simulink model "Sim_Multi"  (R2023a)
settings: Solver=FixedStepAuto  StartTime=0.0  StopTime=20  FixedStep=t_sim  MaxStep=t_control  RelTol=1e-5  EnableMultiTasking=on
InitFcn:
  | %--------------------------------------------------------------------------
  | %% Multirotor Dynamic Simulation Environment for the Testing of GNC Algorithms
  | % This simulation is part of the Master's thesis titled
  | % "A Modular Simulation Environment for the Improved Dynamic Simulation of
  | % Multirotor Unmanned Aerial Vehicles",
  | % submitted to the University of Illinois at Urbana-Champaign in May 2016.
  | % The thesis itself can be found here: http://hdl.handle.net/2142/90660
  | % Jan Vervoorst, vervoors@illinois.edu
  | % University of Illinois 2015/16
  | %--------------------------------------------------------------------------
  | %% Initialization routine for the Simulink simulation file Sim_Multi.slx
  | %--------------------------------------------------------------------------
  | clear all;close all;clc
  | %--------------------------------------------------------------------------
  | t_control = 1/500;          % Controller/state estimation frequency 500Hz [s]
  | t_sim = t_control/2;        % Simulation frequency 1000Hz [s]
  | sim_time = 10.0;            % Duration of simulation [sec]
  | r2d = 180/pi;               % Conversion factor radians to degrees [deg/rad]
  | d2r = pi/180;               % Conversion factor degrees to radians [rad/deg]
  | g = 9.80665;                % Acceleration of gravity [m/s^2]
  | rpm2radpersec = 2*pi/60;    % Conversion factor RPM to rad/sec [rad/(s*rpm)]
  | rho = 1.225;                % Density of air [kg/m^3]
  | %--------------------------------------------------------------------------
  | %%%%%%%%%%%%%%%%%%%%%%%%%%%%%%%%%%%%%%%%%%%%%%%%%%%%%%%%%%%%%%%%%%%%%%%%%%%
  | %               Quad specific configuration parameters                    %
  | %%%%%%%%%%%%%%%%%%%%%%%%%%%%%%%%%%%%%%%%%%%%%%%%%%%%%%%%%%%%%%%%%%%%%%%%%%%
  | % The coordinate system used in this model is defined as follows:
  | % X: pointing forward, Roll axis
  | % Y: pointing to the right, Pitch axis
  | % Z: pointing down, Yaw axis
  | % To define the geometry of the airframe, the following convention is used:
  | % - the base airframe is assumed to be somewhat symmetric
  | % - the CoG for the base airframe coincides with the geometric center in X/Y plane (but is shifted along Z axis)
  | % - the motor arm length in X/Y plane is defined as the distance to the geometric center of the base airframe
  | % - motor thrust is generated at the prop, which is offset a distance (along Z) from the geometric center
  | % - motor thrust vector may be misaligned from purely Z direction, so a set of rotation angles is given for each motor
  | % - real position of CoG is given as a position vector from geometric center
  | % - everything is expressed in body coordinate system described above
  | %%%%%%%%%%%%%%%%%%%%%%%%%%%%%%%%%%%%%%%%%%%%%%%%%%%%%%%%%%%%%%%%%%%%%%%%%%%
  | Noise_flag = 0;                 % Set to 1 for sensor/estimation noise, to 0 for no noise
  | Coriolis_correction = 1;        % Set to 1 to cancel omega x (J*omega) term in control law, 0 if not
  | Dyn_thrust = 1;                 % Set to 1 to engage dynamic thrust effects, to 0 to disengage
  | Blade_flapping = 1;             % Set to 1 to engage blade flapping effects, to 0 to disengage
  | %%%%%%%%%%%%%%%%%%%%%%%%%%%%%%%%
  | % Initial conditions
  | Att_init = [0;0;0] * d2r;       % Initial airframe attitude in Euler angles Roll/Pitch/Yaw for 6DOF block [deg]
  | omega_init = [0;0;0];           % Initial angular rates in Body frame for 6DOF block [rad/s]
  | Vb_init = [0;0;0];              % Initial velocity in Body frame for 6DOF block [m/s]
  | Xi_init = [0;0;0];              % Initial position in Inertial frame for 6DOF block [m]
  | rpm_init = 3104.5025852;        % Initial motor speed [rpm]
  | q_init = rpy2quat(Att_init);    % Compute the initial attitude quaternion
  | R_IB_init = rpy2rot(Att_init);  % Compute the initial rotation matrix R_IB
  | Vi_init = R_IB_init' * Vb_init; % Compute the initial velocity in Inertial axes
  | %%%%%%%%%%%%%%%%%%%%%%%%%%%%%%%%
  | % Parameters for aerodynamic drag computation
  | a = 0.060;                      % Surface area of airframe visible along the Body x axis [m^2]
  | b = 0.060;                      % Surface area of airframe visible along the Body y axis [m^2]
  | c = 0.060;                      % Surface area of airframe visible along the Body z axis [m^2]
  | C_D = 0.40;                     % Drag coefficient [dimensionless]
  | Surface_params = [a;b;c];       % Combine the surface area parameters
  | %%%%%%%%%%%%%%%%%%%%%%%%%%%%%%%%
  | % Parameters for dynamic thrust computation
  | v_h = 4.0;                      % Induced aerodynamic velocity at hover [m/s]
  | kappa = 1.00;                   % Value for induced power factor in hover (chosen to make transition from different states continuous)
  | k1 = -1.125;                    % Empirical values taken from Hoffmann_2011
  | k2 = -1.372;                    % Empirical values taken from Hoffmann_2011
  | k3 = -1.718;                    % Empirical values taken from Hoffmann_2011
  | k4 = -0.655;                    % Empirical values taken from Hoffmann_2011
  | %%%%%%%%%%%%%%%%%%%%%%%%%%%%%%%%
  | % Parameters for blade flapping computation
  | k_a1s = 1.5 / 4.0;              % Gain in linear relationship between wind velocity and flapping angle [deg/(m/s)]
  | k_beta = 0.23;                  % Stiffness of the propeller blades [Nm/rad]
  | %%%%%%%%%%%%%%%%%%%%%%%%%%%%%%%%
  | % Real airframe data
  | CoG_real = [0;0;0.001];         % Location of center of gravity w.r.t. geometric center (in Body axes) [m]
  | mass_real = 0.550;              % Complete airframe mass [kg]
  | Jxx = 0.003960;                 %
  | Jxy = 0;                        %
  | Jxz = 0;                        %
  | Jyx = 0;                        %
  | Jyy = 0.003845;                 % Moment of inertia for multirotor w.r.t center of gravity [kg*m^2]
  | Jyz = 0;                        %
  | Jzx = 0;                        %
  | Jzy = 0;                        %
  | Jzz = 0.007350;                 %
  | J_real = [Jxx Jxy Jxz;Jyx Jyy Jyz;Jzx Jzy Jzz]; % Moment of inertia matrix
  | %%%%%%%%%%%%%%%%%%%%%%%%%%%%%%%%
  | % MotorMatrix_real holds all the information about the actual performance
  | % of each actuator. The data is arranged as one row per motor/prop combo:
  | % 1      : Motor arm angle measured clockwise (looking from above) from the positive X axis (forward direction) [deg]
  | % 2      : Distance of prop/motor in X/Y plane from the geometric center of the airframe [m]
  | % 3      : Distance of prop/motor in Z direction from the geometric center of the airframe [m]
  | % 4      : Direction of prop rotation: -1 for CW, +1 for CCW [unitless]
  | % 5      : Control effectiveness of the actuator (nominally 1.0)
  | % 6      : First-order motor transfer function time constant [sec]
  | % 7..8   : Two coefficients that describe the RPM to thrust [N] transfer function for static conditions [a1 a2]
  | %          Thrust = a1 * RPM + a2 * RPM^2
  | % 9..10  : Two coefficients that describe the RPM to torque [Nm] transfer function for static conditions [b1 b2]
  | %          Torque = b1 * RPM + b2 * RPM^2
  | % 11     : Minimum RPM value of the actuator
  | % 12     : Maximum RPM value of the actuator
  | % 13..15 : Rotations of thrust vector around Body-fixed axes away from nominal direction [deg]
  | %          Nominal direction of thrust vector is [0;0;-1]
  | %          Rotation order from body to motor axes is Yaw/Pitch/Roll (Euler angle sequence (1,2,3))
  | % 16     : Propeller diameter [m]
  | % 17     : Propeller mass [kg]
  | 
  | length1 = 0.170;
  | length2 = 0.170;
  | length3 = 0.170;
  | length4 = 0.170;
  | 
  | MotorMatrix_real = [045 , length1 , -0.028 , -1 , 1.0 , 0.010 , [9.6820 , 0.010872]*1e-5 , [1.4504 , 0.0016312]*1e-6 , 0000 , 6000 , [0.0 , 0.0 , 0.0] , 8*2.54/100 , 11/1000; ...
  |                     135 , length2 , -0.028 , +1 , 1.0 , 0.010 , [9.6820 , 0.010872]*1e-5 , [1.4504 , 0.0016312]*1e-6 , 0000 , 6000 , [0.0 , 0.0 , 0.0] , 8*2.54/100 , 11/1000; ...
  |                     225 , length3 , -0.028 , -1 , 1.0 , 0.010 , [9.6820 , 0.010872]*1e-5 , [1.4504 , 0.0016312]*1e-6 , 0000 , 6000 , [0.0 , 0.0 , 0.0] , 8*2.54/100 , 11/1000; ...
  |                     315 , length4 , -0.028 , +1 , 1.0 , 0.010 , [9.6820 , 0.010872]*1e-5 , [1.4504 , 0.0016312]*1e-6 , 0000 , 6000 , [0.0 , 0.0 , 0.0] , 8*2.54/100 , 11/1000];
  | %%%%%%%%%%%%%%%%%%%%%%%%%%%%%%%%
  | % Nominal airframe data (without disturbance/uncertainties)
  | CoG_nominal = [0;0;0.001];      % Location of center of gravity w.r.t. geometric center (in Body axes) [m]
  | mass_nominal = 0.550;           % Complete airframe mass [kg]
  | Jxx = 0.003960;                 %
  | Jxy = 0;                        %
  | Jxz = 0;                        %
  | Jyx = 0;                        %
  | Jyy = 0.003845;                 % Moment of inertia for multirotor w.r.t center of gravity [kg*m^2]
  | Jyz = 0;                        %
  | Jzx = 0;                        %
  | Jzy = 0;                        %
  | Jzz = 0.007350;                 %
  | J_nominal = [Jxx Jxy Jxz;Jyx Jyy Jyz;Jzx Jzy Jzz]; % Moment of inertia matrix
  | k_torque = 3/200;               % Factor how thrust and induced moment are related (from motor test data)
  | thrust_reserve = 0.10;          % Limit total commanded thrust to 10...90% of max thrust to still allow maneuverability
  | %%%%%%%%%%%%%%%%%%%%%%%%%%%%%%%%
  | % MotorMatrix_nominal holds the nominal information that the controller
  | % assumes about each actuator. Again, the data is arranged as one row per
  | % motor/prop combo:
  | % 1      : Motor arm angle measured clockwise (looking from above) from the positive X axis (forward direction) [deg]
  | % 2      : Distance of prop/motor in X/Y plane from the geometric center of the airframe [m]
  | % 3      : Distance of prop/motor in Z direction from the geometric center of the airframe [m]
  | % 4      : Direction of prop rotation: -1 for CW, +1 for CCW [unitless]
  | % 5      : Control effectiveness of the actuator (nominally 1.0)
  | % 6      : First-order motor transfer function time constant [sec]
  | % 7..8   : Two coefficients that describe the RPM to thrust [N] transfer function for static conditions [a1 a2]
  | %          Thrust = a1 * RPM + a2 * RPM^2
  | % 9..10  : Two coefficients that describe the RPM to torque [Nm] transfer function for static conditions [b1 b2]
  | %          Torque = b1 * RPM + b2 * RPM^2
  | % 11     : Minimum RPM value of the actuator
  | % 12     : Maximum RPM value of the actuator
  | % 13..15 : Rotations of thrust vector around Body-fixed axes away from nominal direction [deg]
  | %          Nominal direction of thrust vector is [0;0;-1]
  | %          Rotation order from body to motor axes is Yaw/Pitch/Roll (Euler angle sequence (1,2,3))
  | % 16     : Propeller diameter [m]
  | % 17     : Propeller mass [kg]
  | MotorMatrix_nominal = [045 , length1 , -0.028 , -1 , 1.0 , 0.010 , [9.6820 , 0.010872]*1e-5 , [1.4504 , 0.0016312]*1e-6 , 0000 , 6000 , [0.0 , 0.0 , 0.0] , 8*2.54/100 , 11/1000; ...
  |                        135 , length2 , -0.028 , +1 , 1.0 , 0.010 , [9.6820 , 0.010872]*1e-5 , [1.4504 , 0.0016312]*1e-6 , 0000 , 6000 , [0.0 , 0.0 , 0.0] , 8*2.54/100 , 11/1000; ...
  |                        225 , length3 , -0.028 , -1 , 1.0 , 0.010 , [9.6820 , 0.010872]*1e-5 , [1.4504 , 0.0016312]*1e-6 , 0000 , 6000 , [0.0 , 0.0 , 0.0] , 8*2.54/100 , 11/1000; ...
  |                        315 , length4 , -0.028 , +1 , 1.0 , 0.010 , [9.6820 , 0.010872]*1e-5 , [1.4504 , 0.0016312]*1e-6 , 0000 , 6000 , [0.0 , 0.0 , 0.0] , 8*2.54/100 , 11/1000];
  | %%%%%%%%%%%%%%%%%%%%%%%%%%%%%%%%%%%%%%%%%%%%%%%%%%%%%%%%%%%%%%%%%%%%%%%%%%%
  | %                          Radio scaling factor                           %
  | %%%%%%%%%%%%%%%%%%%%%%%%%%%%%%%%%%%%%%%%%%%%%%%%%%%%%%%%%%%%%%%%%%%%%%%%%%%
  | % Compute the scaling factor to turn radio throttle command into a thrust value
  | max_thrust = 0;
  | min_thrust = 0;
  | for i = 1:size(MotorMatrix_nominal,1)
  |     max_thrust = max_thrust + (MotorMatrix_nominal(i,7)*MotorMatrix_nominal(i,12)+MotorMatrix_nominal(i,8)*MotorMatrix_nominal(i,12)^2);
  |     min_thrust = min_thrust + (MotorMatrix_nominal(i,7)*MotorMatrix_nominal(i,11)+MotorMatrix_nominal(i,8)*MotorMatrix_nominal(i,11)^2);
  | end
  | thrust_gain = (max_thrust - min_thrust) / 1000;
  | thrust_offset = min_thrust;
  | % %%%%%%%%%%%%%%%%%%%%%%%%%%%%%%%%%%%%%%%%%%%%%%%%%%%%%%%%%%%%%%%%%%%%%%%%%%%
  | % %                   Compute the motor mapping matrix                      %
  | % %%%%%%%%%%%%%%%%%%%%%%%%%%%%%%%%%%%%%%%%%%%%%%%%%%%%%%%%%%%%%%%%%%%%%%%%%%%
  | % % This matrix describes the mapping from body torques to motor thrusts.
  | for i = 1:size(MotorMatrix_nominal,1)
  |     % The vector from nominal center of gravity to nominal location of each propeller
  |     prop_vector(i,1:3) = [abs(MotorMatrix_nominal(i,2)) * [cos(MotorMatrix_nominal(i,1)*d2r);sin(MotorMatrix_nominal(i,1)*d2r)];MotorMatrix_nominal(i,3)] - CoG_nominal;
  |     % The nominal direction in which each motor generates thrust force
  |     thrust_direction(i,1:3) = -[cos(MotorMatrix_nominal(i,13)*d2r)*sin(MotorMatrix_nominal(i,14)*d2r)*cos(MotorMatrix_nominal(i,15)*d2r)+sin(MotorMatrix_nominal(i,13)*d2r)*sin(MotorMatrix_nominal(i,15)*d2r); ...
  |                               cos(MotorMatrix_nominal(i,13)*d2r)*sin(MotorMatrix_nominal(i,14)*d2r)*sin(MotorMatrix_nominal(i,15)*d2r)-sin(MotorMatrix_nominal(i,13)*d2r)*cos(MotorMatrix_nominal(i,15)*d2r); ...
  |                               cos(MotorMatrix_nominal(i,13)*d2r)*cos(MotorMatrix_nominal(i,14)*d2r)];
  |     % The B matrix relates motor thrust to body torques and thrust
  |     % Each column describes one motor/prop. Entries by row 1-4:
  |     % contributions to roll/pitch/yaw torques and thrust, respectively
  | 	B(1:3,i) = cross(prop_vector(i,:)',thrust_direction(i,:)') + k_torque*thrust_direction(i,:)'*MotorMatrix_nominal(i,4);
  |     B(4,i) = 1.0;
  | end
  | % For any airframe with a number of actuators other than four, the B matrix
  | % is nonsquare and therefore taking the regular inverse will not work.
  | % Instead we use the Moore-Penrose pseudoinverse for matrices with linearly
  | % independent rows:
  | MotorMap = B' * inv(B * B');
  | 
  | %%%%%%%%%%%%%%%%%%%%%%%%%%%%%%%%%%%%%%%%%%%%%%%%%%%%%%%%%%%%%%%%%%%%%%%%%%%
  | %              Tuning parameters for the controllers                      %
  | %%%%%%%%%%%%%%%%%%%%%%%%%%%%%%%%%%%%%%%%%%%%%%%%%%%%%%%%%%%%%%%%%%%%%%%%%%%
  | % Controller settings
  | Att_cmd_init = [0;0;0] * d2r;           % Initial attitude command for quaternion strapdown equation initialization in control law
  | MaxRate_cmd = [360;360;120] * d2r;      % Maximum rate command at full stick deflection [rad/s]
  | MaxAtt_cmd = 50 * d2r;                  % Max angle command at full stick deflection [rad]
  | Ref_bw = 10.0;                          % Reference system bandwidth for rate command generation in attitude control
  | %%%%%%%%%%%%%%%%%%%%%%%%%%%%%%%%
  | % Gains for simple PI controller on rates
  | Kp_1  = 15*[1;1;1.5];
  | Ki_1  = 10*[1;1;1.5];
  | Kff_1 = 0.7*[1;1;0.95];
undefined symbols (not defined in the file or in its folder): DiscIntNeverNeededParam, rpy2quat, thrust2rpm
libraries: simulink x20
(part 1 of 4)
settings Model: Creator=JV  LastModifiedBy=divij
settings SolverCC: AlgebraicLoopSolver=TrustRegion
settings DataIOCC: LimitDataPoints=on  SaveFormat=Structure  SignalLoggingSaveFormat=ModelDataLogs  ReturnWorkspaceOutputs=off
settings OptimizationCC: DefaultParameterBehavior=Inlined  UseDivisionForNetSlopeComputation=on  GainParamInheritBuiltInType=on  UseFloatMulNetSlope=on  InlineInvariantSignals=on  ExpressionDepthLimit=2147483647  ZeroExternalMemoryAtStartup=off  ZeroInternalMemoryAtStartup=off  EfficientFloat2IntCast=on  LifeSpan=1  OptimizeDataStoreBuffers=off  BusAssignmentInplaceUpdate=off
settings DebuggingCC: UnderspecifiedInitializationDetection=Classic  SolverPrmCheckMsg=warning  FcnCallInpInsideContextMsg=warning  UnconnectedInputMsg=warning  UnconnectedOutputMsg=warning  UnconnectedLineMsg=warning  StateNameClashWarn=warning  SFUnexpectedBacktrackingDiag=warning  SFNoUnconditionalDefaultTransitionDiag=warning  SFExecutionAtInitializationDiag=none  ArithmeticOperatorsInVariantConditions=warning
settings HardwareCC: ProdBitPerPointer=32  ProdBitPerSizeT=32  ProdBitPerPtrDiffT=32  ProdLargestAtomicFloat=None  ProdIntDivRoundTo=Undefined  ProdEndianess=Unspecified  ProdWordSize=32  ProdHWDeviceType=32-bit Generic
settings ModelReferenceCC: EnableRefExpFcnMdlSchedulingChecks=on  PropagateSignalLabelsOutOfModel=off
settings SFSimCC: SimUseLocalCustomCode=off  MATLABDynamicMemAlloc=off  CustomCodeUndefinedFunction=UseInterfaceOnly
settings RTWCC: PackageGeneratedCodeAndArtifacts=on  GenerateReport=on  RTWUseLocalCustomCode=off  Toolchain=Catkin  BuildConfiguration=Debug  LaunchReport=on  TargetLang=C++
settings CodeAppCC: ForceParamTrailComments=on  EnableCustomComments=on
settings GRTTargetCC: TargetLangStandard=C++11 (ISO)  CombineSignalStateStructs=on  MatFileLogging=off  CodeInterfacePackaging=C++ class  SupportVariableSizeSignals=on  MultiInstanceErrorCode=Warning
settings ConfigComp: CovMetricSettings=dw  CovSaveCumulativeToWorkspaceVar=on  CovSaveSingleToWorkspaceVar=on  CovExternalEMLEnable=off  CovSFcnEnable=off

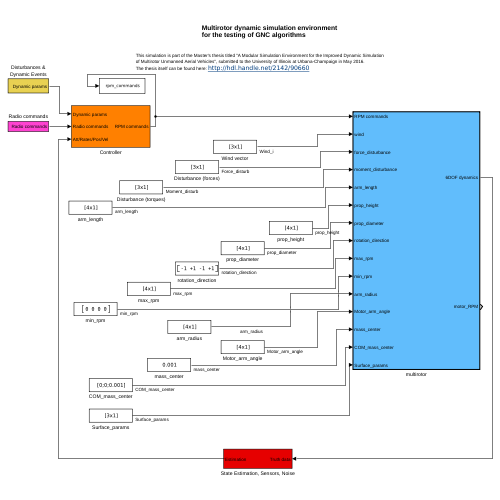
[thumbnail: Simulink's stored preview of the top-level diagram]
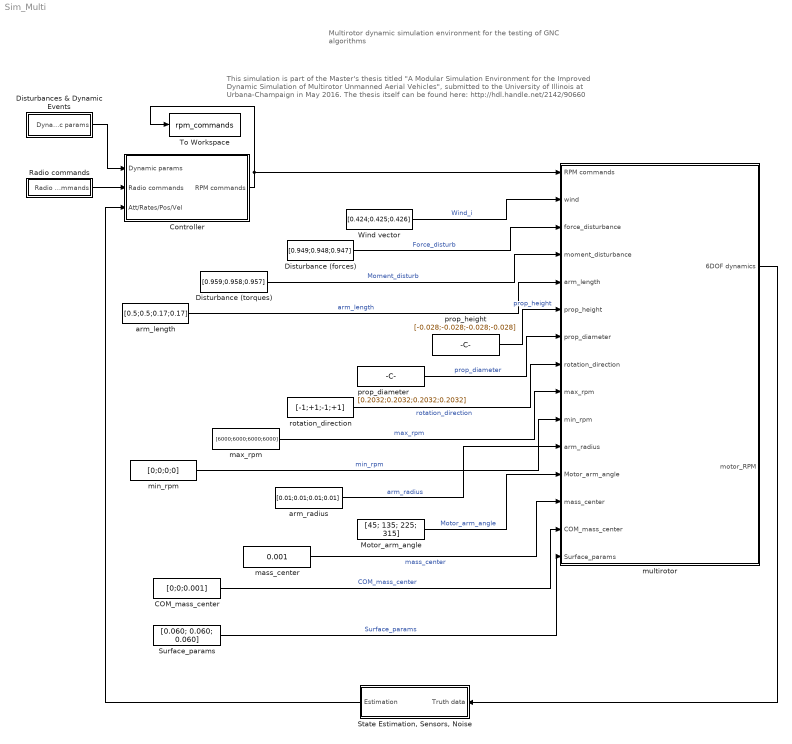
== system Sim_Multi ==
  note: This simulation is part of the Master's thesis titled "A Modular Simulation Environment for the Improved Dynamic Simulation
      | of Multirotor Unmanned Aerial Vehicles", submitted to the University of Illinois at Urbana-Champaign in May 2016.
      | The thesis itself can be found here: http://hdl.handle.net/2142/90660
  note: Multirotor dynamic simulation environment
      | for the testing of GNC algorithms
  COM_mass_center : Constant  Value=[0;0;0.001]
  Controller : Subsystem
  Disturbance (forces) : Constant  Value=[0.949;0.948;0.947]
  Disturbance (torques) : Constant  Value=[0.959;0.958;0.957]
  Disturbances & Dynamic Events : Subsystem
  Motor_arm_angle : Constant  Value=[45; 135; 225; 315]
  Radio commands : Subsystem
  "State Estimation, Sensors, Noise" : Subsystem
  Surface_params : Constant  Value=[0.060; 0.060; 0.060]
  To Workspace : ToWorkspace  VariableName=rpm_commands  SaveFormat=Structure  SampleTime=-1
      settings: Save2DSignal=2-D array (concatenate along first dimension)
  Wind vector : Constant  Value=[0.424;0.425;0.426]
  arm_length : Constant  Value=[0.5;0.5;0.17;0.17]
  arm_radius : Constant  Value=[0.01;0.01;0.01;0.01]
  mass_center : Constant  Value=0.001
  max_rpm : Constant  Value=[6000;6000;6000;6000]
  min_rpm : Constant  Value=[0;0;0;0]
  multirotor : Subsystem  TreatAsAtomicUnit=on
  prop_diameter : Constant  Value=[0.2032;0.2032;0.2032;0.2032]
  prop_height : Constant  Value=[-0.028;-0.028;-0.028;-0.028]
  rotation_direction : Constant  Value=[-1;+1;-1;+1]
  wires:
  multirotor/1(6DOF dynamics) -> "State Estimation, Sensors, Noise"/1(Truth data)
  Radio commands/1(Radio commands) -> Controller/2(Radio commands)
  "State Estimation, Sensors, Noise"/1(Estimation) -> Controller/3(Att/Rates/Pos/Vel)
  Disturbances & Dynamic Events/1(Dynamic params) -> Controller/1(Dynamic params)
  Controller/1(RPM commands) -> To Workspace/1, multirotor/1(RPM commands)
  Wind vector/1 -> multirotor/2(wind)  "Wind_i"
  Disturbance (forces)/1 -> multirotor/3(force_disturbance)  "Force_disturb"
  Disturbance (torques)/1 -> multirotor/4(moment_disturbance)  "Moment_disturb"
  arm_length/1 -> multirotor/5(arm_length)  "arm_length"
  prop_height/1 -> multirotor/6(prop_height)  "prop_height"
  prop_diameter/1 -> multirotor/7(prop_diameter)  "prop_diameter"
  rotation_direction/1 -> multirotor/8(rotation_direction)  "rotation_direction"
  max_rpm/1 -> multirotor/9(max_rpm)  "max_rpm"
  min_rpm/1 -> multirotor/10(min_rpm)  "min_rpm"
  arm_radius/1 -> multirotor/11(arm_radius)  "arm_radius"
  Motor_arm_angle/1 -> multirotor/12(Motor_arm_angle)  "Motor_arm_angle"
  mass_center/1 -> multirotor/13(mass_center)  "mass_center"
  COM_mass_center/1 -> multirotor/14(COM_mass_center)  "COM_mass_center"
  Surface_params/1 -> multirotor/15(Surface_params)  "Surface_params"

== system Sim_Multi/Controller ==
  note: All system parameters used in this block are the nominal parameters
      | that the controller is given about the system.
      | The true parameters of the dynamic system such as mass, inertia,
      | motor mapping matrix, ... may differ from these values.
  Dynamic params : Inport
  Radio commands : Inport  Port=2
  Att/Rates/Pos/Vel : Inport  Port=3
  Controller Structure : Subsystem
  Mapping thrust to rpm and saturation : Subsystem
  Motor mapping : Subsystem
  Reshape : Reshape  OutputDimensionality=Column vector (2-D)
  RPM commands : Outport
  tag scope: RPM_commands=global
  wires:
  Att/Rates/Pos/Vel/1 -> Controller Structure/2(Att/Rates/Pos/Vel)
  Controller Structure/1(Torques/thrust cmd) -> Motor mapping/1(Torques/thrust cmd)
  Radio commands/1 -> Controller Structure/1(Radio commands)
  Reshape/1 -> RPM commands/1
  Dynamic params/1 -> Controller Structure/3(Dynamic params), Mapping thrust to rpm and saturation/2(Dynamic parameters)
  Mapping thrust to rpm and saturation/1(RPM_cmd) -> [RPM_commands], Reshape/1
  Motor mapping/1(Thrust cmds) -> Mapping thrust to rpm and saturation/1(Thrust_cmds)

== system Sim_Multi/Disturbances & Dynamic Events ==
  Bus Creator : BusCreator  Inputs=12
  Constant : Constant  Value=MotorMatrix_real
  Constant1 : Constant  Value=CoG_real
  Constant2 : Constant  Value=mass_real
  Constant3 : Constant  Value=J_real
  Constant4 : Constant  Value=MotorMatrix_nominal
  Constant5 : Constant  Value=CoG_nominal
  Constant6 : Constant  Value=mass_nominal
  Constant7 : Constant  Value=J_nominal
  Disturbance (forces) : Constant  Value=0*[1;1;1]
  Disturbance (torques) : Constant  Value=0*[1;1;1]
  Surface area params : Constant  Value=Surface_params
  Wind vector : Constant  Value=[0;0;0]
  Dynamic params : Outport
  wires:
  Bus Creator/1 -> Dynamic params/1
  Constant/1 -> Bus Creator/1  "MotorMatrix_real"
  Constant1/1 -> Bus Creator/2  "CoG_real"
  Constant2/1 -> Bus Creator/3  "mass_real"
  Constant3/1 -> Bus Creator/4  "J_real"
  Surface area params/1 -> Bus Creator/12  "Surface_params"
  Disturbance (torques)/1 -> Bus Creator/11  "Moment_disturb"
  Disturbance (forces)/1 -> Bus Creator/10  "Force_disturb"
  Wind vector/1 -> Bus Creator/9  "Wind_i"
  Constant4/1 -> Bus Creator/5  "MotorMatrix_nominal"
  Constant5/1 -> Bus Creator/6  "CoG_nominal"
  Constant6/1 -> Bus Creator/7  "mass_nominal"
  Constant7/1 -> Bus Creator/8  "J_nominal"

== system Sim_Multi/Radio commands ==
  Rate Transition : RateTransition  OutPortSampleTime=t_control
  Rate commands : Subsystem
  Radio commands : Outport
  wires:
  Rate commands/1(Rate commands) -> Rate Transition/1
  Rate Transition/1 -> Radio commands/1

== system Sim_Multi/State Estimation, Sensors, Noise ==
  Truth data : Inport
  Rate Transition : RateTransition  OutPortSampleTime=t_control
  Sensor models : Subsystem
  State estimation : Subsystem
  Estimation : Outport
  wires:
  State estimation/1(Att/Pos/Vel/Accel) -> Rate Transition/1
  Sensor models/1(Corrupted) -> State estimation/1(Sensors)
  Truth data/1 -> Sensor models/1(Truth)
  Rate Transition/1 -> Estimation/1

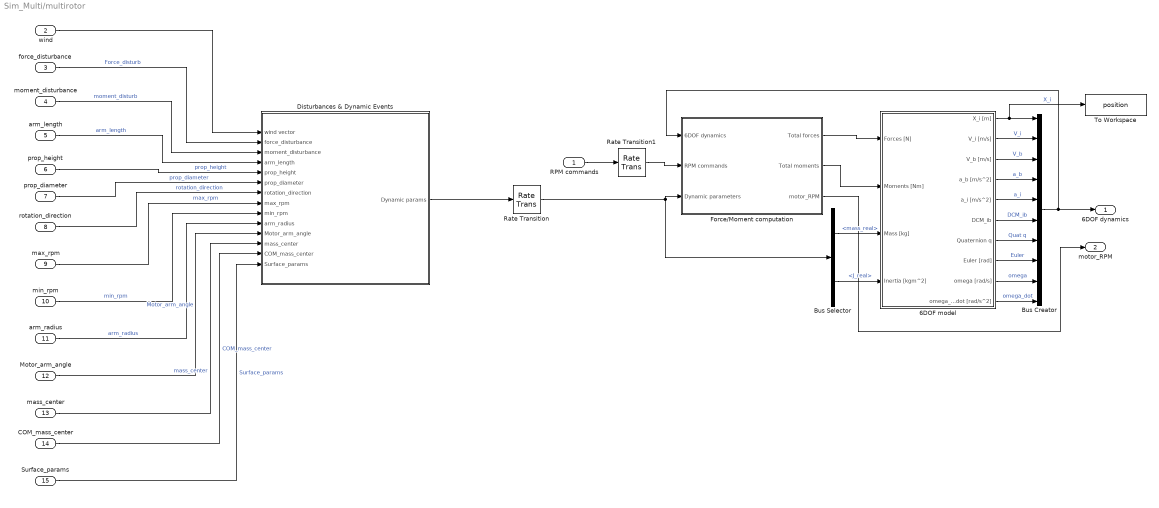
== system Sim_Multi/multirotor ==
  RPM commands : Inport
  wind : Inport  Port=2
  force_disturbance : Inport  Port=3
  moment_disturbance : Inport  Port=4
  arm_length : Inport  Port=5
  prop_height : Inport  Port=6
  prop_diameter : Inport  Port=7
  rotation_direction : Inport  Port=8
  max_rpm : Inport  Port=9
  min_rpm : Inport  Port=10
  arm_radius : Inport  Port=11
  Motor_arm_angle : Inport  Port=12
  mass_center : Inport  Port=13
  COM_mass_center : Inport  Port=14
  Surface_params : Inport  Port=15
  6DOF model : Subsystem
  Bus Creator : BusCreator  Inputs=10
  Bus Selector : BusSelector  OutputSignals=mass_real,J_real
  Disturbances & Dynamic Events : Subsystem
  Force/Moment computation : Subsystem
  Rate Transition : RateTransition  OutPortSampleTime=t_sim
  Rate Transition1 : RateTransition  InitialCondition=rpm_init  OutPortSampleTime=t_sim
  To Workspace : ToWorkspace  VariableName=position  SaveFormat=Structure With Time  SampleTime=-1
      settings: Save2DSignal=2-D array (concatenate along first dimension)
  6DOF dynamics : Outport
  motor_RPM : Outport  Port=2
  wires:
  RPM commands/1 -> Rate Transition1/1
  Bus Creator/1 -> Force/Moment computation/1(6DOF dynamics), 6DOF dynamics/1
  Disturbances & Dynamic Events/1(Dynamic params) -> Rate Transition/1
  6DOF model/1(X_i [m]) -> To Workspace/1, Bus Creator/1  "X_i"
  6DOF model/2(V_i [m/s]) -> Bus Creator/2  "V_i"
  6DOF model/3(V_b [m/s]) -> Bus Creator/3  "V_b"
  6DOF model/4(a_b [m/s^2]) -> Bus Creator/4  "a_b"
  Bus Selector/2 -> 6DOF model/4(Inertia [kgm^2])  "<J_real>"
  Bus Selector/1 -> 6DOF model/3(Mass [kg])  "<mass_real>"
  Force/Moment computation/1(Total forces) -> 6DOF model/1(Forces [N])
  Force/Moment computation/2(Total moments) -> 6DOF model/2(Moments [Nm])
  Rate Transition1/1 -> Force/Moment computation/2(RPM commands)
  Rate Transition/1 -> Force/Moment computation/3(Dynamic parameters), Bus Selector/1
  6DOF model/5(a_i [m/s^2]) -> Bus Creator/5  "a_i"
  6DOF model/6(DCM_ib) -> Bus Creator/6  "DCM_ib"
  6DOF model/7(Quaternion q) -> Bus Creator/7  "Quat q"
  6DOF model/8(Euler [rad]) -> Bus Creator/8  "Euler"
  6DOF model/9(omega [rad/s]) -> Bus Creator/9  "omega"
  6DOF model/10(omega_dot [rad/s^2]) -> Bus Creator/10  "omega_dot"
  force_disturbance/1 -> Disturbances & Dynamic Events/2(force_disturbance)  "Force_disturb"
  moment_disturbance/1 -> Disturbances & Dynamic Events/3(moment_disturbance)  "moment_disturb"
  wind/1 -> Disturbances & Dynamic Events/1(wind vector)
  Force/Moment computation/3(motor_RPM) -> motor_RPM/1
  arm_length/1 -> Disturbances & Dynamic Events/4(arm_length)  "arm_length"
  prop_height/1 -> Disturbances & Dynamic Events/5(prop_height)  "prop_height"
  prop_diameter/1 -> Disturbances & Dynamic Events/6(prop_diameter)  "prop_diameter"
  rotation_direction/1 -> Disturbances & Dynamic Events/7(rotation_direction)  "rotation_direction"
  max_rpm/1 -> Disturbances & Dynamic Events/8(max_rpm)  "max_rpm"
  min_rpm/1 -> Disturbances & Dynamic Events/9(min_rpm)  "min_rpm"
  arm_radius/1 -> Disturbances & Dynamic Events/10(arm_radius)  "arm_radius"
  Motor_arm_angle/1 -> Disturbances & Dynamic Events/11(Motor_arm_angle)  "Motor_arm_angle"
  mass_center/1 -> Disturbances & Dynamic Events/12(mass_center)  "mass_center"
  COM_mass_center/1 -> Disturbances & Dynamic Events/13(COM_mass_center)  "COM_mass_center"
  Surface_params/1 -> Disturbances & Dynamic Events/14(Surface_params)  "Surface_params"

== system Sim_Multi/Controller/Controller Structure ==
  Radio commands : Inport
  Att/Rates/Pos/Vel : Inport  Port=2
  Dynamic params : Inport  Port=3
  Bus Selector : BusSelector  OutputSignals=J_nominal
  Inner-loop control only : Subsystem
  Torques/thrust cmd : Outport
  tag scope: J_control=global
  wires:
  Dynamic params/1 -> Bus Selector/1
  Bus Selector/1 -> [J_control]  "<J_nominal>"
  Radio commands/1 -> Inner-loop control only/2(Radio commands)
  Att/Rates/Pos/Vel/1 -> Inner-loop control only/1(Att/Rates/Pos/Vel)
  Inner-loop control only/1(Control out) -> Torques/thrust cmd/1

== system Sim_Multi/Controller/Mapping thrust to rpm and saturation ==
  Thrust_cmds : Inport
  Dynamic parameters : Inport  Port=2
  Bus Selector1 : BusSelector  OutputSignals=MotorMatrix_nominal
  For Each Subsystem : Subsystem  TreatAsAtomicUnit=on
  Rate Transition : RateTransition  OutPortSampleTime=t_control
  RPM_cmd : Outport
  wires:
  For Each Subsystem/1(RPM_cmd_sat) -> Rate Transition/1
  Dynamic parameters/1 -> Bus Selector1/1
  Bus Selector1/1 -> For Each Subsystem/2(MotorMatrix_nominal)  "<MotorMatrix_nominal>"
  Rate Transition/1 -> RPM_cmd/1
  Thrust_cmds/1 -> For Each Subsystem/1(Thrust_cmds)

== system Sim_Multi/Controller/Motor mapping ==
  note: Overall thrust command is limited to a range
      | of 10...90% of max thrust to still allow room
      | for torque demands needed for maneuvering
  note: The motor mapping matrix used here to transform body axis torque commands
      | into thrust commands for each motor is populated with the nominal arm length
      | and motor position information that the controller thinks are correct, not the
      | actual values used in the true dynamics computation block.
  Torques/thrust cmd : Inport
  Constant1 : Constant  Value=MotorMap
  Demux : Demux  Outputs=[3 1]
  Matrix Multiply1 : Product  Multiplication=Matrix(*)
  Max thrust limit : Subsystem
  Min thrust limit : Subsystem
  Mux : Mux  Inputs=2
  Rate Transition : RateTransition  OutPortSampleTime=t_control
  Saturation Dynamic : simulink/Discontinuities/Saturation Dynamic  OutMin=[]  OutMax=[]  OutDataTypeStr=Inherit: Same as second input  OutDataType=fixdt(1, 16)  OutScaling=2^-10  DoSatur=off
  Thrust cmds : Outport
  wires:
  Constant1/1 -> Matrix Multiply1/1
  Rate Transition/1 -> Thrust cmds/1  "These are thrust demands to each motor"
  Matrix Multiply1/1 -> Rate Transition/1
  Torques/thrust cmd/1 -> Demux/1
  Demux/2 -> Saturation Dynamic/2
  Min thrust limit/1(Out1) -> Saturation Dynamic/3
  Max thrust limit/1(Out1) -> Saturation Dynamic/1
  Saturation Dynamic/1 -> Mux/2
  Demux/1 -> Mux/1
  Mux/1 -> Matrix Multiply1/2

== system Sim_Multi/Radio commands/Rate commands ==
  note: The signal magnitude for the throttle should be
      | in a range of [0,1000]
  Filter : Subsystem
  Mux : Mux  Inputs=3
  Mux1 : Mux  Inputs=2
  Pitch rate signal : Subsystem
  Rate Transition : RateTransition  OutPortSampleTime=t_control
  Roll rate signal : Subsystem
  Throttle value : Constant  Value=299.9916292904752
  Yaw rate signal : Subsystem
  Rate commands : Outport
  wires:
  Filter/2(theta_dot filtered) -> Mux/2
  Mux1/1 -> Rate commands/1
  Filter/3(psi_dot filtered) -> Mux/3
  Filter/1(phi_dot filtered) -> Mux/1
  Roll rate signal/1(phi) -> Filter/1(Roll rate)
  Mux/1 -> Rate Transition/1
  Pitch rate signal/1(theta) -> Filter/2(Pitch rate)
  Yaw rate signal/1(psi) -> Filter/3(Yaw rate)
  Throttle value/1 -> Mux1/2
  Rate Transition/1 -> Mux1/1

== system Sim_Multi/State Estimation, Sensors, Noise/Sensor models ==
  note: The available sensor outputs are body rates and body accelerations.
      | In the simple case, noise is added to the rate and accel outputs of the 6DOF block to 'simulate' sensor output.
  Truth : Inport
  Acc noise : Subsystem
  Bus Creator : BusCreator  Inputs=9
  Bus Selector : BusSelector  OutputSignals=a_b,omega
  Bus Selector1 : BusSelector  OutputSignals=X_i,V_i,V_b,DCM_ib,Quat q,Euler,omega_dot
  Gain : Gain
  Gain1 : Gain
  Gyro noise : Subsystem
  Noisy acc : Scope
  Noisy omega : Scope
  Sum : Sum
  Sum1 : Sum
  Corrupted : Outport
  wires:
  Truth/1 -> Bus Selector/1, Bus Selector1/1
  Bus Creator/1 -> Corrupted/1
  Sum/1 -> Noisy omega/1, Gain/1  "omega"
  Sum1/1 -> Noisy acc/1, Gain1/1  "a_b"
  Bus Selector1/1 -> Bus Creator/1  "<X_i>"
  Bus Selector1/2 -> Bus Creator/2  "<V_i>"
  Bus Selector1/3 -> Bus Creator/3  "<V_b>"
  Acc noise/1(Noise) -> Sum1/1
  Bus Selector/1 -> Sum1/2  "<a_b>"
  Gain1/1 -> Bus Creator/4  "a_b"
  Bus Selector1/4 -> Bus Creator/5  "<DCM_ib>"
  Bus Selector1/5 -> Bus Creator/6  "<Quat q>"
  Bus Selector1/6 -> Bus Creator/7  "<Euler>"
  Gyro noise/1(Noise) -> Sum/2
  Bus Selector/2 -> Sum/1  "<omega>"
  Gain/1 -> Bus Creator/8  "omega"
  Bus Selector1/7 -> Bus Creator/9  "<omega_dot>"

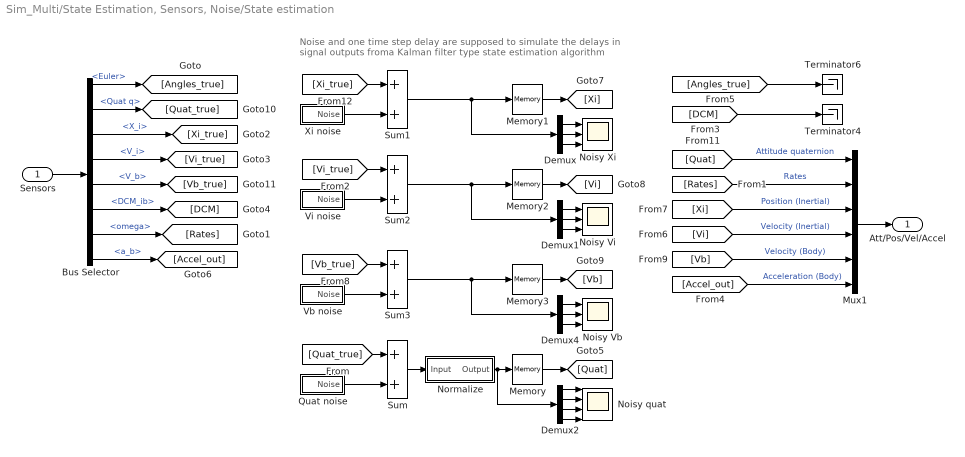
== system Sim_Multi/State Estimation, Sensors, Noise/State estimation ==
  note: Noise and one time step delay are supposed to simulate the delays
      | in signal outputs froma Kalman filter type state estimation algorithm
  Sensors : Inport
  Bus Selector : BusSelector  OutputSignals=Euler,Quat q,X_i,V_i,V_b,DCM_ib,omega,a_b
  Demux : Demux  Outputs=3
  Demux1 : Demux  Outputs=3
  Demux2 : Demux
  Demux4 : Demux  Outputs=3
  Memory : Memory  InitialCondition=q_init
  Memory1 : Memory  InitialCondition=Xi_init
  Memory2 : Memory  InitialCondition=Vi_init
  Memory3 : Memory  InitialCondition=Vi_init
  Mux1 : Mux  Inputs=6
  Noisy Vb : Scope  NumInputPorts=3
  Noisy Vi : Scope  NumInputPorts=3
  Noisy Xi : Scope  NumInputPorts=3
  Noisy quat : Scope  NumInputPorts=4
  Normalize : Subsystem
  Quat noise : Subsystem
  Sum{,1..3} (4 alike) : Sum
  Terminator4 : Terminator
  Terminator6 : Terminator
  Vb noise : Subsystem
  Vi noise : Subsystem
  Xi noise : Subsystem
  Att/Pos/Vel/Accel : Outport
  wires:
  Sensors/1 -> Bus Selector/1
  Bus Selector/3 -> [Xi_true]  "<X_i>"
  Bus Selector/4 -> [Vi_true]  "<V_i>"
  Bus Selector/6 -> [DCM]  "<DCM_ib>"
  Bus Selector/7 -> [Rates]  "<omega>"
  Bus Selector/8 -> [Accel_out]  "<a_b>"
  Bus Selector/1 -> [Angles_true]  "<Euler>"
  [Quat] -> Mux1/1  "Attitude quaternion"
  [Rates] -> Mux1/2  "Rates"
  Bus Selector/2 -> [Quat_true]  "<Quat q>"
  [DCM] -> Terminator4/1
  [Angles_true] -> Terminator6/1
  Sum/1 -> Normalize/1(Input)
  Quat noise/1(Noise) -> Sum/2
  [Quat_true] -> Sum/1
  Normalize/1(Output) -> Demux2/1, Memory/1
  Memory/1 -> [Quat]
  Xi noise/1(Noise) -> Sum1/2
  Sum1/1 -> Demux/1, Memory1/1
  Memory1/1 -> [Xi]
  [Xi_true] -> Sum1/1
  Vi noise/1(Noise) -> Sum2/2
  Memory2/1 -> [Vi]
  [Vi_true] -> Sum2/1
  [Xi] -> Mux1/3  "Position (Inertial)"
  [Vi] -> Mux1/4  "Velocity (Inertial)"
  Mux1/1 -> Att/Pos/Vel/Accel/1
  Sum2/1 -> Demux1/1, Memory2/1
  Demux/1 -> Noisy Xi/1
  Demux/2 -> Noisy Xi/2
  Demux/3 -> Noisy Xi/3
  Demux1/1 -> Noisy Vi/1
  Demux1/2 -> Noisy Vi/2
  Demux1/3 -> Noisy Vi/3
  Demux2/1 -> Noisy quat/1
  Demux2/2 -> Noisy quat/2
  Demux2/3 -> Noisy quat/3
  Demux2/4 -> Noisy quat/4
  Vb noise/1(Noise) -> Sum3/2
  Memory3/1 -> [Vb]
  [Vb_true] -> Sum3/1
  Sum3/1 -> Demux4/1, Memory3/1
  Demux4/1 -> Noisy Vb/1
  Demux4/2 -> Noisy Vb/2
  Demux4/3 -> Noisy Vb/3
  Bus Selector/5 -> [Vb_true]  "<V_b>"
  [Vb] -> Mux1/5  "Velocity (Body)"
  [Accel_out] -> Mux1/6  "Acceleration (Body)"

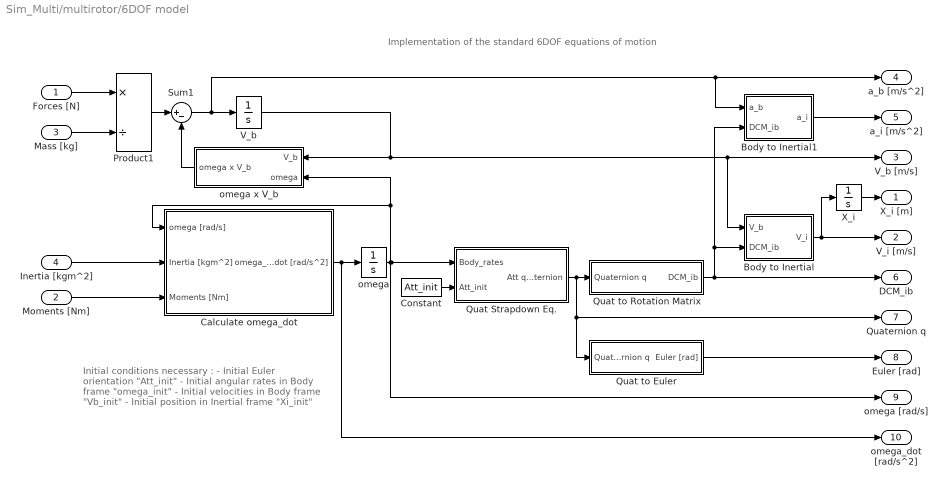
== system Sim_Multi/multirotor/6DOF model ==
  note: Implementation of the standard 6DOF equations of motion
  note: Initial conditions necessary :
      | - Initial Euler orientation "Att_init"
      | - Initial angular rates in Body frame "omega_init"
      | - Initial velocities in Body frame "Vb_init"
      | - Initial position in Inertial frame "Xi_init"
  Forces [N] : Inport
  Moments [Nm] : Inport  Port=2
  Mass [kg] : Inport  Port=3
  Inertia [kgm^2] : Inport  Port=4
  Body to Inertial : Subsystem
  Body to Inertial1 : Subsystem
  Calculate omega_dot : Subsystem
  Constant : Constant  Value=Att_init
  Product1 : Product  Inputs=*/  SaturateOnIntegerOverflow=on  OutDataTypeStr=Inherit: Same as first input
  Quat Strapdown Eq. : Subsystem
  Quat to Euler : Subsystem
  Quat to Rotation Matrix : Subsystem
  Sum1 : Sum  Inputs=|+-  SaturateOnIntegerOverflow=on
  V_b : Integrator  InitialCondition=Vb_init
  X_i : Integrator  InitialCondition=Xi_init
  omega : Integrator  InitialCondition=omega_init
  omega x V_b : Subsystem
  X_i [m] : Outport
  V_i [m/s] : Outport  Port=2
  V_b [m/s] : Outport  Port=3
  a_b [m/s^2] : Outport  Port=4
  a_i [m/s^2] : Outport  Port=5
  DCM_ib : Outport  Port=6
  Quaternion q : Outport  Port=7
  Euler [rad] : Outport  Port=8
  omega [rad/s] : Outport  Port=9
  omega_dot [rad/s^2] : Outport  Port=10
  wires:
  Forces [N]/1 -> Product1/1
  Mass [kg]/1 -> Product1/2
  Product1/1 -> Sum1/1
  omega x V_b/1(omega x V_b) -> Sum1/2
  V_b/1 -> V_b [m/s]/1, Body to Inertial/1(V_b), omega x V_b/1(V_b)
  Inertia [kgm^2]/1 -> Calculate omega_dot/2(Inertia [kgm^2])
  Moments [Nm]/1 -> Calculate omega_dot/3(Moments [Nm])
  Calculate omega_dot/1(omega_dot [rad/s^2]) -> omega_dot [rad/s^2]/1, omega/1
  omega/1 -> Calculate omega_dot/1(omega [rad/s]), omega x V_b/2(omega), omega [rad/s]/1, Quat Strapdown Eq./1(Body_rates)
  Quat Strapdown Eq./1(Att quaternion) -> Quat to Euler/1(Quaternion q), Quaternion q/1, Quat to Rotation Matrix/1(Quaternion q)
  Quat to Euler/1(Euler [rad]) -> Euler [rad]/1
  Body to Inertial/1(V_i) -> V_i [m/s]/1, X_i/1
  X_i/1 -> X_i [m]/1
  Constant/1 -> Quat Strapdown Eq./2(Att_init)
  Quat to Rotation Matrix/1(DCM_ib) -> Body to Inertial1/2(DCM_ib), Body to Inertial/2(DCM_ib), DCM_ib/1
  Body to Inertial1/1(a_i) -> a_i [m/s^2]/1
  Sum1/1 -> V_b/1, a_b [m/s^2]/1, Body to Inertial1/1(a_b)

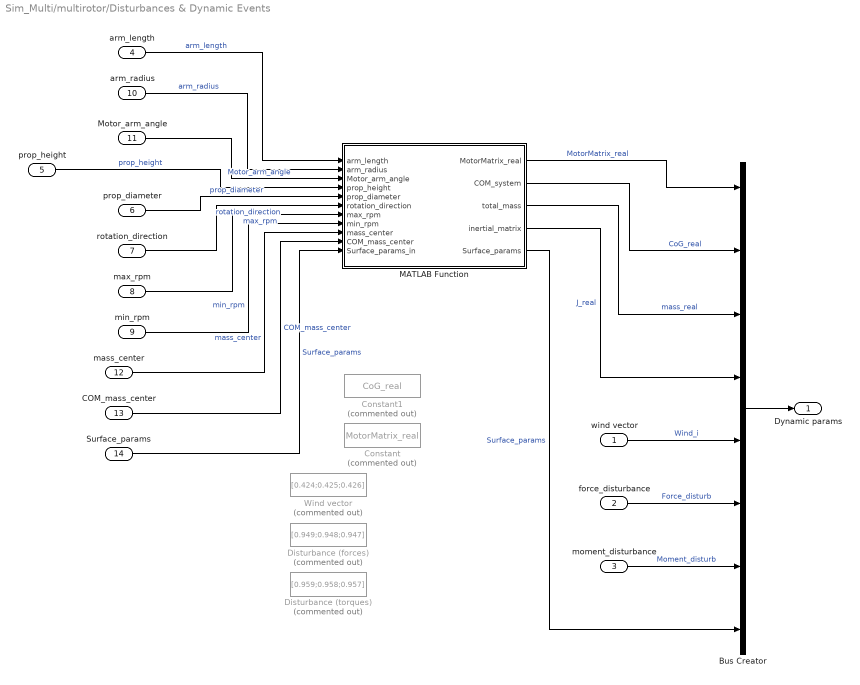
== system Sim_Multi/multirotor/Disturbances & Dynamic Events ==
  wind vector : Inport
  force_disturbance : Inport  Port=2
  moment_disturbance : Inport  Port=3
  arm_length : Inport  Port=4
  prop_height : Inport  Port=5
  prop_diameter : Inport  Port=6
  rotation_direction : Inport  Port=7
  max_rpm : Inport  Port=8
  min_rpm : Inport  Port=9
  arm_radius : Inport  Port=10
  Motor_arm_angle : Inport  Port=11
  mass_center : Inport  Port=12
  COM_mass_center : Inport  Port=13
  Surface_params : Inport  Port=14
  Bus Creator : BusCreator  Inputs=8
  Constant : Constant  Commented=on  Value=MotorMatrix_real
  Constant1 : Constant  Commented=on  Value=CoG_real
  Disturbance (forces) : Constant  Commented=on  Value=[0.949;0.948;0.947]
  Disturbance (torques) : Constant  Commented=on  Value=[0.959;0.958;0.957]
  MATLAB Function : MATLAB Function  TreatAsAtomicUnit=on
  Wind vector : Constant  Commented=on  Value=[0.424;0.425;0.426]
  Dynamic params : Outport
  wires:
  Bus Creator/1 -> Dynamic params/1
  MATLAB Function/1(MotorMatrix_real) -> Bus Creator/1  "MotorMatrix_real"
  MATLAB Function/2(COM_system) -> Bus Creator/2  "CoG_real"
  MATLAB Function/3(total_mass) -> Bus Creator/3  "mass_real"
  MATLAB Function/4(inertial_matrix) -> Bus Creator/4  "J_real"
  MATLAB Function/5(Surface_params) -> Bus Creator/8  "Surface_params"
  moment_disturbance/1 -> Bus Creator/7  "Moment_disturb"
  force_disturbance/1 -> Bus Creator/6  "Force_disturb"
  wind vector/1 -> Bus Creator/5  "Wind_i"
  arm_length/1 -> MATLAB Function/1(arm_length)  "arm_length"
  prop_height/1 -> MATLAB Function/4(prop_height)  "prop_height"
  prop_diameter/1 -> MATLAB Function/5(prop_diameter)  "prop_diameter"
  rotation_direction/1 -> MATLAB Function/6(rotation_direction)  "rotation_direction"
  max_rpm/1 -> MATLAB Function/7(max_rpm)  "max_rpm"
  min_rpm/1 -> MATLAB Function/8(min_rpm)  "min_rpm"
  arm_radius/1 -> MATLAB Function/2(arm_radius)  "arm_radius"
  Motor_arm_angle/1 -> MATLAB Function/3(Motor_arm_angle)  "Motor_arm_angle"
  mass_center/1 -> MATLAB Function/9(mass_center)  "mass_center"
  COM_mass_center/1 -> MATLAB Function/10(COM_mass_center)  "COM_mass_center"
  Surface_params/1 -> MATLAB Function/11(Surface_params_in)  "Surface_params"

== system Sim_Multi/multirotor/Force//Moment computation ==
  note: Computation of all forces and moments acting on the airframe
  6DOF dynamics : Inport
  RPM commands : Inport  Port=2
  Dynamic parameters : Inport  Port=3
  Bus Selector : BusSelector  OutputSignals=Force_disturb,Moment_disturb
  Compute aerodynamic drag of the airframe in Body axes : Subsystem
  Compute force of gravity in Body axes : Subsystem
  Forces and moments generated by spinning propellers : Subsystem
  Sum{,1..3} (4 alike) : Sum  Inputs=|++
  Total forces : Outport
  Total moments : Outport  Port=2
  motor_RPM : Outport  Port=3
  wires:
  RPM commands/1 -> Forces and moments generated by spinning propellers/1(RPM_commands)
  6DOF dynamics/1 -> Forces and moments generated by spinning propellers/3(6DOF dynamics), Compute aerodynamic drag of the airframe in Body axes/1(6DOF dynamics), Compute force of gravity in Body axes/1(6DOF dynamics)
  Forces and moments generated by spinning propellers/2(Motor forces) -> Sum/1
  Compute force of gravity in Body axes/1(Gravity force) -> Sum/2
  Dynamic parameters/1 -> Bus Selector/1, Compute aerodynamic drag of the airframe in Body axes/2(Dynamic parameters), Compute force of gravity in Body axes/2(Dynamic parameters), Forces and moments generated by spinning propellers/2(Dynamic parameters)
  Bus Selector/1 -> Sum1/2  "<Force_disturb>"
  Bus Selector/2 -> Sum2/2  "<Moment_disturb>"
  Forces and moments generated by spinning propellers/1(Motor moments) -> Sum2/1
  Sum/1 -> Sum3/1
  Sum3/1 -> Sum1/1
  Compute aerodynamic drag of the airframe in Body axes/1(Drag force) -> Sum3/2
  Sum2/1 -> Total moments/1
  Sum1/1 -> Total forces/1
  Forces and moments generated by spinning propellers/3(motor_RPM) -> motor_RPM/1

== system Sim_Multi/Controller/Controller Structure/Inner-loop control only ==
  note: The output of the inner-loop controller is always
      | a set of three commanded torques around the
      | Body axes, roll/pitch/yaw, and an overall thrust
      | command.
      | This is independent of what the structure of the
      | multirotor airframe is assumed to be.
  Att/Rates/Pos/Vel : Inport
  Radio commands : Inport  Port=2
  Conversion stick values to rate commands : Subsystem
  Demux : Demux  Outputs=[4 3 3 3 3 3]
  PI Rate controller : Subsystem
  Terminator{,1..4} (5 alike) : Terminator
  Control out : Outport
  wires:
  Att/Rates/Pos/Vel/1 -> Demux/1
  Demux/3 -> Terminator/1  "Xi"
  Demux/4 -> Terminator1/1  "Vi"
  Demux/5 -> Terminator2/1  "Vb"
  Demux/6 -> Terminator3/1  "a_b"
  Radio commands/1 -> Conversion stick values to rate commands/1(Sticks/Throttle cmd)
  PI Rate controller/1(Control/Throttle out) -> Control out/1
  Demux/2 -> PI Rate controller/2(Rate_est)
  Conversion stick values to rate commands/1(Rates/Throttle cmd) -> PI Rate controller/1(Rates/Throttle cmd)
  Demux/1 -> Terminator4/1

== system Sim_Multi/Controller/Mapping thrust to rpm and saturation/For Each Subsystem ==
  note: The thrust commands from the controller are turned into RPM commands by solving the
      | nominal (quadratic) rpm to thrust equations for RPM.
      | These min and max RPM values are then saturated using the nominal min and max RPM
      | values given for the particular motor/propeller combination.
  Thrust_cmds : Inport  Partition=on  PartitionDimension=1  PartitionWidth=1  PartitionOffset=0
  MotorMatrix_nominal : Inport  Port=2  Partition=on  PartitionDimension=1  PartitionWidth=1  PartitionOffset=0
  For Each : ForEach  DisableCoverage=on
  MATLAB Function : MATLAB Function  TreatAsAtomicUnit=on
  Mux : Mux  Inputs=2
  Saturation Dynamic : simulink/Discontinuities/Saturation Dynamic  OutMin=[]  OutMax=[]  OutDataTypeStr=Inherit: Same as second input  OutDataType=fixdt(1, 16)  OutScaling=2^-10  DoSatur=off
  Saturation limit: no negative thrust : Saturate  UpperLimit=inf  LowerLimit=0
  Selector1 : Selector  InputPortWidth=17  IndexOptions=Index vector (dialog)  Indices=[11]  OutputSizes=1
  Selector2 : Selector  InputPortWidth=17  IndexOptions=Index vector (dialog)  Indices=[12]  OutputSizes=1
  Selector3 : Selector  InputPortWidth=17  IndexOptions=Index vector (dialog)  Indices=[7 8]  OutputSizes=1
  thrust2rpm : MATLABFcn  Commented=on  MATLABFcn=thrust2rpm(u)  OutputDimensions=1
  RPM_cmd_sat : Outport  ConcatenationDimension=1
  wires:
  Selector3/1 -> Mux/1  "Thrust params a1 and a2"
  Thrust_cmds/1 -> Saturation limit: no negative thrust/1
  Mux/1 -> MATLAB Function/1(thrust_input)
  MATLAB Function/1(rpm_output) -> Saturation Dynamic/2  "Commanded RPM value for each motor"
  Selector2/1 -> Saturation Dynamic/1  "Nominal max RPM"
  Selector1/1 -> Saturation Dynamic/3  "Nominal min RPM"
  Saturation Dynamic/1 -> RPM_cmd_sat/1
  MotorMatrix_nominal/1 -> Selector1/1, Selector2/1, Selector3/1
  Saturation limit: no negative thrust/1 -> Mux/2

== system Sim_Multi/Controller/Motor mapping/Max thrust limit ==
  Constant : Constant  Value=max_thrust
  Constant2 : Constant  Value=min_thrust
  Gain : Gain  Gain=thrust_reserve
  Sum : Sum  Inputs=|+-
  Sum1 : Sum  Inputs=+-|
  Out1 : Outport
  wires:
  Constant/1 -> Sum1/1, Sum/1
  Sum1/1 -> Out1/1
  Constant2/1 -> Sum/2
  Sum/1 -> Gain/1
  Gain/1 -> Sum1/2

== system Sim_Multi/Controller/Motor mapping/Min thrust limit ==
  Constant : Constant  Value=max_thrust
  Constant2 : Constant  Value=min_thrust
  Gain : Gain  Gain=thrust_reserve
  Sum : Sum  Inputs=|+-
  Sum1 : Sum  Inputs=|++
  Out1 : Outport
  wires:
  Constant/1 -> Sum/1
  Sum1/1 -> Out1/1
  Constant2/1 -> Sum1/2, Sum/2
  Sum/1 -> Gain/1
  Gain/1 -> Sum1/1

== system Sim_Multi/Radio commands/Rate commands/Filter ==
  Roll rate : Inport
  Pitch rate : Inport  Port=2
  Yaw rate : Inport  Port=3
  Transfer Fcn{1..6} (6 alike) : TransferFcn  Denominator=[.01 1]
  phi_dot filtered : Outport
  theta_dot filtered : Outport  Port=2
  psi_dot filtered : Outport  Port=3
  wires:
  Transfer Fcn6/1 -> Transfer Fcn1/1
  Transfer Fcn2/1 -> Transfer Fcn3/1
  Transfer Fcn4/1 -> Transfer Fcn5/1
  Yaw rate/1 -> Transfer Fcn2/1
  Transfer Fcn3/1 -> psi_dot filtered/1
  Pitch rate/1 -> Transfer Fcn4/1
  Transfer Fcn5/1 -> theta_dot filtered/1
  Roll rate/1 -> Transfer Fcn6/1
  Transfer Fcn1/1 -> phi_dot filtered/1

== system Sim_Multi/Radio commands/Rate commands/Pitch rate signal ==
  note: The signal magnitude for the pitch channel should be at most 1.
      | It then gets scaled by a factor of 500 to simulate a PWM output
      | range of [-500,500]
  Add1 : Sum  Inputs=+++
  Add2 : Sum  Inputs=+++
  Constant : Constant  Value=0
  Gain : Gain
  Gain1 : Gain  Gain=0.1
  Gain2 : Gain  Gain=500
  Manual Switch : ManualSwitch  CurrentSetting=0
  Manual Switch1 : ManualSwitch
  Step1 : Step  SampleTime=0
  Step2 : Step  Time=2  After=-2  SampleTime=0
  Step3 : Step  Time=3.5  SampleTime=0
  Step4 : Step  Time=4.5  After=-2  SampleTime=0
  Step5 : Step  Time=5.5  SampleTime=0
  Step6 : Step  Time=3  SampleTime=0
  theta : Outport
  wires:
  Add1/1 -> Gain/1
  Step3/1 -> Add1/1
  Step4/1 -> Add1/2
  Step5/1 -> Add1/3
  Gain2/1 -> theta/1
  Gain/1 -> Manual Switch/1
  Add2/1 -> Gain1/1
  Step1/1 -> Add2/1
  Step2/1 -> Add2/2
  Step6/1 -> Add2/3
  Gain1/1 -> Manual Switch/2
  Manual Switch/1 -> Manual Switch1/1
  Constant/1 -> Manual Switch1/2
  Manual Switch1/1 -> Gain2/1

== system Sim_Multi/Radio commands/Rate commands/Roll rate signal ==
  note: The signal magnitude for the roll channel should be at most 1.
      | It then gets scaled by a factor of 500 to simulate a PWM output
      | range of [-500,500]
  Add : Sum  Inputs=+++
  Constant : Constant  Value=0
  Gain : Gain  Gain=0.1
  Gain2 : Gain  Gain=500
  Manual Switch : ManualSwitch
  Manual Switch1 : ManualSwitch
  Step : Step  Time=0.5  SampleTime=0
  Step1 : Step  Time=1.5  After=-2  SampleTime=0
  Step2 : Step  Time=2.5  SampleTime=0
  Step3 : Step  Time=0.5  SampleTime=0
  phi : Outport
  wires:
  Step/1 -> Add/1
  Step1/1 -> Add/2
  Step2/1 -> Add/3
  Add/1 -> Gain/1
  Gain2/1 -> phi/1
  Gain/1 -> Manual Switch/1
  Manual Switch/1 -> Manual Switch1/1
  Manual Switch1/1 -> Gain2/1
  Constant/1 -> Manual Switch1/2
  Step3/1 -> Manual Switch/2

== system Sim_Multi/Radio commands/Rate commands/Yaw rate signal ==
  note: The signal magnitude for the yaw channel should be at most 1.
      | It then gets scaled by a factor of 500 to simulate a PWM output
      | range of [-500,500]
  Add1 : Sum  Inputs=+++
  Add2 : Sum  Inputs=+++
  Constant : Constant  Value=0
  Gain : Gain  Gain=0.2
  Gain1 : Gain  Gain=0.2
  Gain2 : Gain  Gain=500
  Manual Switch : ManualSwitch  CurrentSetting=0
  Manual Switch1 : ManualSwitch  CurrentSetting=0
  Step1 : Step  Time=2  SampleTime=0
  Step2 : Step  Time=3  After=-2  SampleTime=0
  Step3 : Step  Time=4  SampleTime=0
  Step6 : Step  Time=6.5  SampleTime=0
  Step7 : Step  Time=7.5  After=-2  SampleTime=0
  Step8 : Step  Time=8.5  SampleTime=0
  psi : Outport
  wires:
  Step6/1 -> Add2/1
  Step7/1 -> Add2/2
  Step8/1 -> Add2/3
  Add2/1 -> Gain1/1
  Gain2/1 -> psi/1
  Step1/1 -> Add1/1
  Step2/1 -> Add1/2
  Step3/1 -> Add1/3
  Add1/1 -> Gain/1
  Gain/1 -> Manual Switch/2
  Manual Switch/1 -> Manual Switch1/1
  Manual Switch1/1 -> Gain2/1
  Constant/1 -> Manual Switch1/2
  Gain1/1 -> Manual Switch/1

== system Sim_Multi/State Estimation, Sensors, Noise/Sensor models/Acc noise ==
  Band-Limited White Noise : simulink/Sources/Band-Limited White Noise  Cov=t_sim*57.3*57.3/10000  Ts=t_sim  seed=[25341]
  Constant : Constant  Value=Noise_flag
  Constant1 : Constant  Value=0
  Gain1 : Gain  Gain=0.1
  Gain2 : Gain  Gain=0.08
  Integrator : Integrator
  Sum1 : Sum  Inputs=++|
  Switch : Switch  Criteria=u2 > Threshold  SaturateOnIntegerOverflow=off  InputSameDT=off
  Uniform Random Number : UniformRandomNumber  Minimum=-.001  Maximum=.001  Seed=657  SampleTime=t_sim
  Noise : Outport
  wires:
  Band-Limited White Noise/1 -> Gain2/1
  Uniform Random Number/1 -> Integrator/1
  Integrator/1 -> Gain1/1
  Switch/1 -> Noise/1
  Constant/1 -> Switch/2
  Constant1/1 -> Switch/3
  Gain2/1 -> Sum1/1
  Gain1/1 -> Sum1/2
  Sum1/1 -> Switch/1

== system Sim_Multi/State Estimation, Sensors, Noise/Sensor models/Gyro noise ==
  Band-Limited White Noise : simulink/Sources/Band-Limited White Noise  Cov=t_sim*57.3*57.3/10000  Ts=t_sim  seed=[23341]
  Constant : Constant  Value=Noise_flag
  Constant1 : Constant  Value=0
  Gain1 : Gain  Gain=0.1
  Gain2 : Gain  Gain=0.07
  Integrator : Integrator
  Sum1 : Sum  Inputs=++|
  Switch : Switch  Criteria=u2 > Threshold  SaturateOnIntegerOverflow=off  InputSameDT=off
  Uniform Random Number : UniformRandomNumber  Minimum=-.001  Maximum=.001  Seed=338  SampleTime=t_sim
  Noise : Outport
  wires:
  Band-Limited White Noise/1 -> Gain2/1
  Uniform Random Number/1 -> Integrator/1
  Integrator/1 -> Gain1/1
  Switch/1 -> Noise/1
  Constant/1 -> Switch/2
  Constant1/1 -> Switch/3
  Gain2/1 -> Sum1/1
  Gain1/1 -> Sum1/2
  Sum1/1 -> Switch/1
